simulink subsystem "ElectricalID_6ph"  (R2021b)
settings: Solver=VariableStepAuto  StartTime=0.0  StopTime=10.0  RelTol=1e-3
libraries: Subchart_Step_Response x6
settings Model: Creator=valen  LastModifiedBy=valen

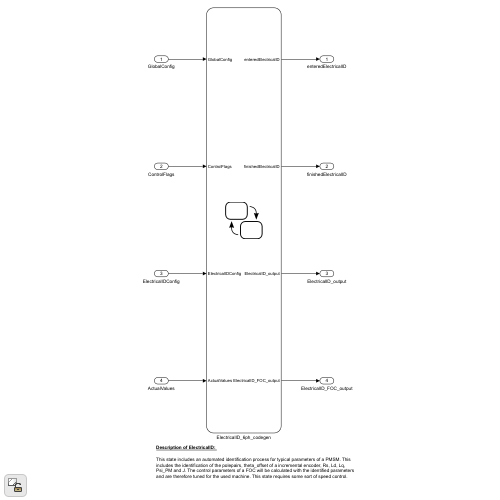
[thumbnail: Simulink's stored preview of the top-level diagram]
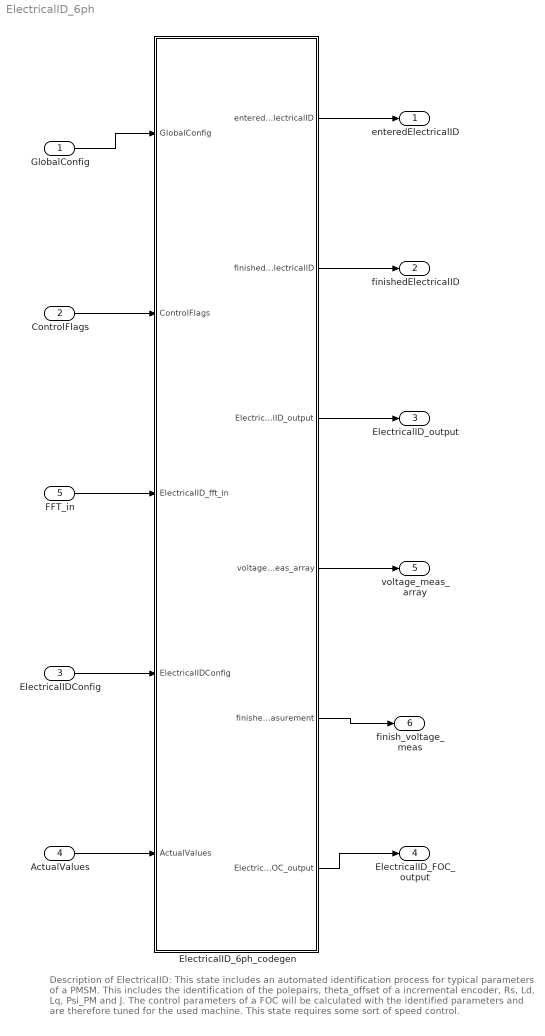
== system ElectricalID_6ph ==
  note: Description of ElectricalID:
      |
      | This state includes an automated identification process for typical parameters of a PMSM. This includes the identification of the polepairs, theta_offset of a incremental encoder, Rs, Ld, Lq, Psi_PM and J. The control parameters of a FOC will be calculated with the identified parameters and are therefore tuned for the used machine. This state requires some sort of speed control.
  GlobalConfig : Inport
  ControlFlags : Inport  Port=2
  ElectricalIDConfig : Inport  Port=3
  ActualValues : Inport  Port=4
  FFT_in : Inport  Port=5  OutDataTypeStr=Bus: uz_ParaID_ElectricalID_fft_in_t
  ElectricalID_6ph_codegen : Stateflow chart
      settings: PortSchema="{\"entries\":[{\"content\":{\"sides\":[{\"content\":{\"connectorIds\":[\"In3\",\"In4\",\"In5\",\"In1\",\"In2\"]},\"type\":\"ConnectorPlacement.EquallySpacedRectSide\",\"uuid\":\"f0ac0bcf-14d9-46a0-98b5-cf926ef17a03\"},{\"content\":{\"connectorIds\":[\"Out1\",\"Out2\",\"Out4\",\"Out5\",\"Out6\",\"Out3\"],\"side\":\"RIGHT\"},\"type\":\"ConnectorPlacement.EquallySpacedRectSide\",\"uuid\":\"3432f655-d87e-4f4a-bc13-594c8277a670\"},{\"content\":{\"connectorIds\":[],\"side\":\"TOP\"},\"type\":\"ConnectorPlacement.EquallySpacedRectSide\",\"uuid\":\"598e67a2-ee08-4059-aaa7-0b5cb688c228\"}]},\"type\":\"ConnectorPlacement.EquallySpacedConnector\",\"uuid\":\"e19c3dd0-4872-4ea8-9ebd-fc7e1d9ddc42\"}],\"packageUris\":[\"http://schema.mathworks.com/mf0/Connector/R2020b\"],\"version\":\"1.0\"}"
  enteredElectricalID : Outport
  finishedElectricalID : Outport  Port=2
  ElectricalID_output : Outport  Port=3
  ElectricalID_FOC_output : Outport  Port=4
  voltage_meas_array : Outport  Port=5
  finish_voltage_meas : Outport  Port=6
  wires:
  ElectricalID_6ph_codegen/3(ElectricalID_FOC_output) -> ElectricalID_FOC_output/1
  ElectricalID_6ph_codegen/4(ElectricalID_output) -> ElectricalID_output/1
  ElectricalID_6ph_codegen/2(finishedElectricalID) -> finishedElectricalID/1
  ControlFlags/1 -> ElectricalID_6ph_codegen/4(ControlFlags)
  ElectricalIDConfig/1 -> ElectricalID_6ph_codegen/1(ElectricalIDConfig)
  ActualValues/1 -> ElectricalID_6ph_codegen/2(ActualValues)
  ElectricalID_6ph_codegen/1(enteredElectricalID) -> enteredElectricalID/1
  GlobalConfig/1 -> ElectricalID_6ph_codegen/3(GlobalConfig)
  FFT_in/1 -> ElectricalID_6ph_codegen/5(ElectricalID_fft_in)
  ElectricalID_6ph_codegen/5(voltage_meas_array) -> voltage_meas_array/1
  ElectricalID_6ph_codegen/6(finished_voltage_measurement) -> finish_voltage_meas/1

== stateflow chart ElectricalID_6ph/ElectricalID_6ph_codegen ==
  settings: updateMethod=DISCRETE  sampleTime=1/d_f_states
  note: PMSM identification
  state ElectricalID
    entry:
    initParams;
    ElectricalID_FOC_output.activeState = uint16(100);
    enteredElectricalID=boolean(1);
    during:
    state waitLock
      entry:
      ElectricalID_FOC_output.activeState = uint16(140);
    state findDutyCycle
      entry:
      ElectricalID_FOC_output.activeState = uint16(110);
      if(ElectricalIDConfig.dutyCyc > 0.0)%Checks if a manual value for the DutyCycle was set
      DutyCycle = single(ElectricalIDConfig.dutyCyc);
      DC_valid = boolean(1);
      else
      DutyCycle = single(0.01);%Starting DC
      DC_valid = boolean(0);
      end
      counter = uint32(1); %starts with 1, so that the DutyCylce_mod function wont be entered
      %during the fist cycle through the state
      during:
      if(DC_valid==0)
      ElectricalID_output.PWM_Switch_0 = single(DutyCycle);%Set DC
      if(counter < uint32(0.4/GlobalConfig.sampleTimeISR))%Wait several time for step response to rise
      counter = counter +1;
      elseif(counter >= uint32(0.4/GlobalConfig.sampleTimeISR) &&....
      counter < uint32(0.5/GlobalConfig.sampleTimeISR))%record current - WHY NOW?
      counter = counter +1;
      ia_sum=ia_sum+single(ActualValues.i_abc_6ph.a1);%integral of current - WHY?
      elseif(counter == uint32(0.5/GlobalConfig.sampleTimeISR))%endtime
      DutyCycle_mod(abs(ia_sum*(GlobalConfig.sampleTimeISR/0.1)));%exec fct
      counter  = uint32(1);
      ia_sum = single(0.0);
      end
      end
      exit:
      ref_amplitude = single(DutyCycle*ActualValues.V_DC);
      ElectricalID_output.PWM_Switch_0 = single(0);
    state waitSetRPM
      entry:
      ElectricalID_FOC_output.activeState = uint16(150);
      ElectricalID_output.enable_TriState = boolean([1 1 1]);
      ElectricalID_output.enable_TriState_set_2 = boolean([1 1 1]);
      f_cutoff = cutoff_frequency(GlobalConfig.voltage_measurement_Rp,GlobalConfig.voltage_measurement_Rs,GlobalConfig.voltage_measurement_C);
      setpoint_rpm = f_cutoff/single(highest_order)/ElectricalID_output.PMSM_parameters.polePairs*single(60);
      setpoint_rpm = correct_setpoint(setpoint_rpm,GlobalConfig.ratSpeed);
    state measure_induced_voltage
      entry:
      ElectricalID_FOC_output.activeState = uint16(151);
      counter = uint32(1);
      during:
      if(counter<=10000)
      voltage_meas_array(counter-1) = ActualValues.v_abc_6ph.a1;
      counter = counter + 1;
      else
      finished_voltage_measurement = true;
      end
      exit:
      counter = uint32(1);
      ElectricalID_output.psi_pm = ElectricalID_fft_in.psi_pm_amplitude;
      ElectricalID_output.psi_pm_angle = ElectricalID_fft_in.psi_pm_angle;
      ElectricalID_output.PMSM_parameters.Psi_PM_Vs = ElectricalID_output.psi_pm(1);
    state Subchart_Step_Response5
    state Subchart_Step_Response
    state Subchart_Step_Response1
    state Subchart_Step_Response2
    state stop 	%state 10.1
      entry:
      ElectricalID_FOC_output.activeState = uint16(160);
      ElectricalID_FOC_output.n_ref_FOC = single(0);
      ElectricalID_FOC_output.resetIntegrator = boolean(1);
      during:counter = counter +1;
    state alignRotor_d_on
      entry:
      ElectricalID_FOC_output.activeState = uint16(120);
      counter = uint32(1);
      during:
      DutyCycle_filt = single(single(counter)*GlobalConfig.sampleTimeISR*2);
      if(DutyCycle_filt > 1)
      DutyCycle_filt = single(1.0);
      end
      ElectricalID_output.PWM_Switch_0 = single(DutyCycle*DutyCycle_filt);
      counter  = counter +1;
      exit:
      ElectricalID_output = ResetDutyCycle(ElectricalID_output);
    state Subchart_Step_Response3
    state rotorInertiaEstimation
      entry:
      ElectricalID_FOC_output.enableFOC_speed = boolean(0);
      ElectricalID_FOC_output.enableFOC_current = boolean(1);
      counter = uint32(1);
      ElectricalID_FOC_output.resetIntegrator = boolean(0);
      ElectricalID_FOC_output.activeState = uint16(161);
      wait_count = uint32(3/GlobalConfig.sampleTimeISR);
      during:
      ElectricalID_FOC_output.i_dq_ref.q = SinusGenerator(ElectricalIDConfig.goertzlTorque,....
      ElectricalIDConfig.goertzlFreq,GlobalConfig.sampleTimeISR);
      if(counter > wait_count && counter < (wait_count+501))
      measArray1(counter-wait_count) = ActualValues.i_dq.q;
      i_est(counter-wait_count) = ActualValues.omega_m;
      end
      counter = counter + 1;
      exit:
      goertzel;
    state Subchart_Step_Response4
    state alignRotor_d_off
      entry:
      counter = uint32(1);
      ElectricalID_output.PWM_Switch_0 = single(0);
      ElectricalID_FOC_output.activeState = uint16(121);
      during:
      counter  = counter +1;
      exit:
      ElectricalID_output.thetaOffset = ActualValues.theta_m;
    state endState
      entry:
      counter = uint32(1);
      ElectricalID_FOC_output.activeState = uint16(162);
      ElectricalID_FOC_output.resetIntegrator=boolean(1);
      during:
      counter = counter + 1;
    state waitAccept
      entry:
      ElectricalID_FOC_output.activeState = uint16(148);
      if(ElectricalIDConfig.identLq ==  0)
      ElectricalID_output.inductances_6ph.q=ElectricalID_output.inductances_6ph.d;
      ElectricalID_output.resistances_6ph.q=ElectricalID_output.resistances_6ph.d;
      end
      ElectricalID_output.PMSM_parameters.Ld_Henry = ElectricalID_output.inductances_6ph.d;
      ElectricalID_output.PMSM_parameters.Lq_Henry = ElectricalID_output.inductances_6ph.q;
      ElectricalID_output.PMSM_parameters.R_ph_Ohm = ElectricalID_output.resistances_6ph.d;
    state waitState 	%do nothing
      entry:
      counter = uint32(1);
      ElectricalID_FOC_output.enableFOC_current = boolean(0);
      ElectricalID_FOC_output.activeState = uint16(170);
      % recalculate speed controller using psiPM and J
      Kp_n_loc = Kp_iq_loc/(ElectricalID_output.PMSM_parameters.Lq_Henry*dampingFactor*...
      GlobalConfig.PMSM_config.polePairs*3.0/2.0*ElectricalID_output.PMSM_parameters.Psi_PM_Vs/....
      ElectricalID_output.PMSM_parameters.J_kg_m_squared);
      Ki_n_loc = (Kp_iq_loc * Kp_iq_loc)/( ElectricalID_output.PMSM_parameters.Lq_Henry * ....
      ElectricalID_output.PMSM_parameters.Lq_Henry * dampingFactor * dampingFactor * dampingFactor * ....
      GlobalConfig.PMSM_config.polePairs*3.0/2.0*ElectricalID_output.PMSM_parameters.Psi_PM_Vs/....
      ElectricalID_output.PMSM_parameters.J_kg_m_squared);
      ElectricalID_FOC_output.Kp_n_out = Kp_n_loc;
      ElectricalID_FOC_output.Ki_n_out = Ki_n_loc;
      during:
      counter = counter + 1;
      exit:
      finishedElectricalID=boolean(1);
      enteredElectricalID=boolean(0);
      reset_FOC_output;
    (default) -> findDutyCycle
    alignRotor_d_off -> waitLock : [one_sec_transition_counter == counter]
    waitLock -> Subchart_Step_Response [order 2] : [ElectricalIDConfig.identLq ==  0 && GlobalConfig.ACCEPT == 1]
    waitLock -> Subchart_Step_Response5 [order 1] : [GlobalConfig.ACCEPT == 1&&ElectricalIDConfig.identLq == 1]
    waitSetRPM -> measure_induced_voltage : [GlobalConfig.ACCEPT==1&&ActualValues.omega_m>5]
    1046 -> Subchart_Step_Response : {ElectricalID_output.inductances_6ph.q=L_est;
        | ElectricalID_output.resistances_6ph.q=R_est;}
    measure_induced_voltage -> stop 	%state 10.1 : [ElectricalID_fft_in.finished_flag]
    1041 -> Subchart_Step_Response1 : {ElectricalID_output.inductances_6ph.d=L_est;
        | ElectricalID_output.resistances_6ph.d=R_est;}
    waitAccept -> waitSetRPM : [GlobalConfig.ACCEPT==1]
    1042 -> Subchart_Step_Response2 : {ElectricalID_output.inductances_6ph.x=L_est;
        | ElectricalID_output.resistances_6ph.x=R_est;}
    findDutyCycle -> alignRotor_d_on : [DC_valid == 1]
    1043 -> Subchart_Step_Response3 : {ElectricalID_output.inductances_6ph.y=L_est;
        | ElectricalID_output.resistances_6ph.y=R_est;}
    stop 	%state 10.1 -> rotorInertiaEstimation : [one_sec_transition_counter == counter && ActualValues.omega_m==single(0)]
    1044 -> Subchart_Step_Response4 : {ElectricalID_output.inductances_6ph.z1=L_est;
        | ElectricalID_output.resistances_6ph.z1=R_est;}
    alignRotor_d_on -> alignRotor_d_off : [one_sec_transition_counter == counter]
    1045 -> waitAccept : {ElectricalID_output.inductances_6ph.z2=L_est;
        | ElectricalID_output.resistances_6ph.z2=R_est}
    rotorInertiaEstimation -> endState : [counter == (wait_count+513)]
    endState -> waitState 	%do nothing : [one_sec_transition_counter == counter]
  state Waiting
    entry:
    %wait for activation of
    %ElectricalID
    %donothing
  state calculatePIcontroller 	%state6.0 [commented out]
    entry:
    ElectricalID_FOC_output.activeState = uint16(149);
    ElectricalID_FOC_output = ControllerParameter(ElectricalID_FOC_output,...
    bandwidthCurrentControl,ElectricalID_output.PMSM_parameters,dampingFactor,psiOverJ);
  Waiting -> ElectricalID [order 1] : [ControlFlags.startElectricalID==1 &&....
      |  GlobalConfig.Reset==0 && GlobalConfig.ACCEPT==1]
  (default) -> Waiting
  Waiting -> Waiting [order 2] : [GlobalConfig.Reset==1]
      | {finishedElectricalID=boolean(0);
      | enteredElectricalID=boolean(0);
      | initParams;}
  waitState 	%do nothing -> Waiting : [one_sec_transition_counter == counter]
  ElectricalID -> Waiting : [GlobalConfig.Reset==1 || GlobalConfig.ElectricalID==0 ||....
      |  GlobalConfig.enableParameterID==0]
      | {enteredElectricalID=boolean(0);initParams;}
  data: ia_reg_in function_input; setpoint function_input; ratSpeed function_input; out function_output; Rp function_input; Rs function_input; C function_input; out function_output; f_cutoff local single size=1; highest_order local uint16 size=1; setpoint_rpm local single size=1; R_est function_output; L_est function_output; activeState function_output; R_est function_output; L_est function_output; activeState function_output; R_est function_output; L_est function_output; activeState function_output; R_est function_output; L_est function_output; activeState function_output; R_est function_output; L_est function_output; activeState function_output; Amp function_input; Freq function_input; sampleTime function_input; y function_output; R_est function_output; L_est function_output; activeState function_output; n_filt local single size=1 =single(0.0); n_ref_old local single size=1 =single(0.0); repetitionCounter local uint32 size=1 =uint32(0); dutyCycAdj local single size=1 =single(0.0); counter local uint32 size=1; k local single size=1; dp local single size=[2,1]; Ndata local uint16 size=1; Nparams local uint16 size=1; DutyCycle_filt local single size=1 =single(0.0); R_corr local single size=1; bandwidthCurrentControl local; dampingFactor local; psiOverJ local; Kp_n_loc local; Ki_n_loc local; Ki_id_loc local; Kp_id_loc local; Ki_iq_loc local; Kp_iq_loc local; meas_sum local single; omega_sum local; om_con local; ia_sum local; J2 local; enteredElectricalID output boolean size=1; finishedElectricalID output boolean size=1; ElectricalIDConfig input Bus: uz_ParaID_ElectricalIDConfig_t size=1; ElectricalID_FOC_output output Bus: uz_ParaID_Controller_Parameters_output_t size=1; ActualValues input Bus: uz_ParaID_ActualValues_t; GlobalConfig input Bus: uz_ParaID_GlobalConfig_t; ControlFlags input Bus: uz_ParaID_ControlFlags_t; d local single size=[2048,1]; DutyCycle local single; ElectricalID_output output Bus: uz_ParaID_ElectricalID_output_t size=1; wait_count local; one_sec_transition_counter local; ref_amplitude local single size=1; measArray1 local; i_est local; R_est local single size=1 =single(0); L_est local single size=1 =single(0); DC_valid local boolean size=1; ElectricalID_fft_in input Bus: uz_ParaID_ElectricalID_fft_in_t size=1; voltage_meas_array output single size=10000; finished_voltage_measurement output boolean size=1
  data ref_amplitude settings: description=Reference amplitude
  data DC_valid settings: description=|
      | Flag: Duty Cycle is valid.
      | Is set by either finding a proper Duty Cycle or setting a Duty Cycle manually
  function DutyCycle_mod(ia_reg_in):
    | function DutyCycle_mod(ia_reg_in)
    | 
    | mean_ia_reg=mean(ia_reg_in);
    | %determines if the mean value is below the step-response current limit
    | if(mean_ia_reg < 0.5*GlobalConfig.ratCurrent)%Current limit for step response  
    | 	DC_valid=boolean(0);    
    | else
    |     DC_valid=boolean(1);
    | end
    |    
    | if(DC_valid == 0)
    | 	%Increases the DutyCycle by 0.5% every 0.5 second, if the step response
    | 	%is below the current limit
    | 	DutyCycle = DutyCycle + 0.005; %Simulation 0.001 | Real 0.005
    | end
    | end
  function out = correct_setpoint(setpoint,ratSpeed):
    | function out = correct_setpoint(setpoint,ratSpeed)   
    | %correct_setpoint corrects the requested rpm
    | %   ties the rpm to rated speed if its higher or rounds it to nearest
    | %   hundred
    | %% function:
    |     % if corrected_setpoint_rpm is larger than n_ref set it to n_ref
    |     if(setpoint>ratSpeed)
    |         out = ratSpeed;
    |     % round setpoint down to nearest 100 
    |     else 
    |         out = round(setpoint/100)*100;
    |         % substract 100 if setpoint was rounded up
    |         if(out>setpoint)
    |             out = out - 100;
    |         end
    |     end    
    | end
  function out = cutoff_frequency(Rp,Rs,C):
    | function out = cutoff_frequency(Rp,Rs,C)
    | %cutoff_frequency determines cutoff frequency for given filter
    | %   uses filter configuration with 2R and a C
    | %% function:
    |     resistance = Rp*Rs/(Rp+Rs);
    |     out = 1/(2*pi*resistance*C);
    | end
  function goertzel:
    | function goertzel
    | 
    | % goertzel algorithm for J calculation
    | 
    | % calculate momentum from i_q
    | for k=single(1):single(500)
    | d(k) = 1.5*GlobalConfig.PMSM_config.polePairs*ElectricalID_output.PMSM_parameters.Psi_PM_Vs*measArray1(k);
    | end
    |  
    | % goertzel
    | ISR_factor = single(0.0001 / GlobalConfig.sampleTimeISR); %Adjusts the k-factor for different ISR frequencys
    | k = single(2.0 / ISR_factor);   % coefficient number of the spectrum (40Hz)
    | N = 500;       % length of input signal
    | 
    | %Precalculation of constants
    | A = 2*pi*k/N;
    | B = 2*cos(A);
    | C = exp(-j*A);
    | %State variables
    | s0 = single(0.0);
    | s1 = single(0.0);
    | s2 = single(0.0);
    | 
    | %Main loop for M
    | for i = 1:N %N multiplications, 2N additions
    | s0 = d(i) +B*s1-s2; %corresponds to (16)
    | s2 = s1;
    | s1 = s0;
    | end
    | 
    | %Finalizing calculations for M
    | s0 = B*s1-s2; %corresponds to (16) with zero input; 1 multiplication and 1 addition
    | Xg = s0-s1*C %corresponds to (17); 4 multiplications and 3 additions
    | 
    | %Reset state variables
    | s0 = single(0.0);
    | s1 = single(0.0);
    | s2 = single(0.0);
    | 
    | %Main loop for omega_m
    | for i = 1:N %N multiplications, 2N additions
    | s0 = i_est(i) +B*s1-s2; %corresponds to (16)
    | s2 = s1;
    | s1 = s0;
    | end
    | 
    | %Finalizing calculations for omega_m
    | s0 = B*s1-s2; %corresponds to (16) with zero input; 1 multiplication and 1 addition
    | Yg = s0-s1*C %corresponds to (17); 4 multiplications and 3 additions
    | 
    | 
    | 
    | % calculate value of transfer function 
    | Gg = Yg/Xg;
    | % calculate J from Gg
    | ElectricalID_output.PMSM_parameters.J_kg_m_squared = single(abs(1/(Gg*j*2*pi*40))); %without damping
  function y = SinusGenerator(Amp, Freq, sampleTime):
    | function y = SinusGenerator(Amp, Freq, sampleTime)
    | %#codegen
    | 
    | persistent sineCounter;
    | 
    | if isempty(sineCounter)
    |     sineCounter = uint32(0); %initialize
    |     u = single(0);
    | end
    |     u = single(Amp*sin(2*pi*single(Freq)*single(sineCounter)*sampleTime));
    |     sineCounter = sineCounter + 1;
    |     if(sineCounter == uint32(1/(single(Freq)*sampleTime)))
    |         sineCounter = uint32(0);
    |     end
    |    
    | 
    | y = single(u);
  function initParams:
    | function initParams
    | 
    | %This is used instead of "after(1.0,sec) to ensure the same transition time
    | %independelty of the sampletime in the c-code
    | one_sec_transition_counter = uint32(1/GlobalConfig.sampleTimeISR);
    | % initialize variables
    | Ki_n_loc            = single(0.0);
    | Kp_n_loc            = single(0.0);
    | n_filt              = single(0.0);
    | n_ref_old           = single(0.0);
    | repetitionCounter   = uint32(0);
    | dutyCycAdj          = single(0.0);
    | counter 			= uint32(1);
    | Kp_iq_loc           = single(0.0);
    | Ki_iq_loc           = single(0.0);
    | Kp_id_loc           = single(0.0);
    | Ki_id_loc           = single(0.0);
    | DutyCycle_filt      = single(0.0);
    | measArray1			= single(zeros(1024,1));
    | meas_sum            = single(zeros(2,1));%used for Friction Id
    | J2                  = single(zeros(256,5));
    | thetaOffset         = single(0.0);
    | Vstep               = single(zeros(205,1));
    | DutyCycle           = single(0.0);
    | omega_sum           = single(0);
    | om_con              = boolean(0);
    | ia_sum              = single(0);
    | ia_valid            = boolean(0);
    | DC_manual           = boolean(0);
    | 
    | %Outputs
    | ElectricalID_FOC_output.Ki_n_out                    = single(0.0);
    | ElectricalID_FOC_output.Ki_iq_out                   = single(0.0);
    | ElectricalID_FOC_output.Ki_id_out                   = single(0.0);
    | ElectricalID_FOC_output.Kp_n_out                    = single(0.0);
    | ElectricalID_FOC_output.Kp_iq_out                   = single(0.0);
    | ElectricalID_FOC_output.Kp_id_out                   = single(0.0);
    | ElectricalID_FOC_output.n_ref_FOC                   = single(0.0);
    | ElectricalID_FOC_output.i_dq_ref.d                  = single(0.0);
    | ElectricalID_FOC_output.i_dq_ref.q                  = single(0.0);
    | ElectricalID_FOC_output.i_dq_ref.zero               = single(0.0);
    | ElectricalID_FOC_output.enableFOC_speed             = boolean(0);
    | ElectricalID_FOC_output.enableFOC_current           = boolean(0);
    | ElectricalID_FOC_output.resetIntegrator             = boolean(0);
    | ElectricalID_FOC_output.activeState                 = uint16(0);
    | finishedElectricalID= boolean(0);
    | 
    | ElectricalID_output.PWM_Switch_0                        = single(0.0);
    | ElectricalID_output.PWM_Switch_2                        = single(0.0);
    | ElectricalID_output.PWM_Switch_4                        = single(0.0);
    | ElectricalID_output.PWM_Switch_a2                        = single(0.0);
    | ElectricalID_output.PWM_Switch_b2                        = single(0.0);
    | ElectricalID_output.PWM_Switch_c2                        = single(0.0);
    | ElectricalID_output.enable_TriState                     = boolean(zeros(1,3)); %0 = TriState off, 1 = TriState on   
    | ElectricalID_FOC_output.activeState                     = uint16(0);
    | ElectricalID_output.thetaOffset                         = single(0.0);
    | ElectricalID_output.PMSM_parameters.R_ph_Ohm            = single(0.0);
    | ElectricalID_output.PMSM_parameters.Ld_Henry            = single(0.0);
    | ElectricalID_output.PMSM_parameters.Lq_Henry            = single(0.0);
    | ElectricalID_output.PMSM_parameters.Psi_PM_Vs           = single(0.0);
    | ElectricalID_output.PMSM_parameters.polePairs           = GlobalConfig.PMSM_config.polePairs;
    | ElectricalID_output.PMSM_parameters.J_kg_m_squared      = single(0.0);
    | enteredElectricalID                                     = boolean(0);
    | 
    | % initialize variables for Levenberg-Marquardt
    | d        			= single(zeros(2048,1));
    | dp      			= single(zeros(2,1));
    | e       			= single(0);
    | e_lm  				= single(0);
    | H 					= single(zeros(2,2));
    | i_est 				= single(zeros(2048,1));
    | it 					= uint16(0);
    | J 					= single(zeros(2048,2));
    | k 					= single(0);
    | L0 					= single(0);
    | L_est   			= single(0);
    | L_lm 				= single(0);
    | Ndata  				= uint16(512);
    | Nparams 			= uint16(2);
    | n_iters 			= uint16(100);
    | R0 					= single(0);
    | R_est 				= single(0);
    | R_lm 				= single(0);
    | V0 					= single(0);
    | lambda  			= single(0.01);
    | updateJ 			= boolean(1);
    | 
    | % initialize varaibles for PMSM parameters
    | R_corr              = single(0.000); %0.060
    | 
    | % variables for controller calculation
    | bandwidthCurrentControl = single(1000); 
    | dampingFactor           = single(10.0);
    | psiOverJ                = single(5000);
    | 
    | end
  function reset_FOC_output:
    | function reset_FOC_output
    | 
    | %Outputs
    | ElectricalID_FOC_output.n_ref_FOC           = single(0.0);
    | ElectricalID_FOC_output.i_dq_ref.d          = single(0.0);
    | ElectricalID_FOC_output.i_dq_ref.q          = single(0.0);
    | ElectricalID_FOC_output.i_dq_ref.zero       = single(0.0);
    | ElectricalID_FOC_output.enableFOC_speed     = boolean(0);
    | ElectricalID_FOC_output.enableFOC_current   = boolean(0);
    | ElectricalID_FOC_output.resetIntegrator     = boolean(0);
    | ElectricalID_FOC_output.activeState         = uint16(0);
    | TwoMassID_FOC_output.Kp_id_out              = single(Kp_id_loc);
    | TwoMassID_FOC_output.Kp_iq_out              = single(Kp_iq_loc);
    | TwoMassID_FOC_output.Kp_n_out               = single(Kp_n_loc);
    | TwoMassID_FOC_output.Ki_id_out              = single(Ki_id_loc);
    | TwoMassID_FOC_output.Ki_iq_out              = single(Ki_iq_loc);
    | TwoMassID_FOC_output.Ki_n_out               = single(Ki_n_loc);
    | end
